simulink model "CS637Assignment1_1"  (R2022a)
settings: Solver=VariableStepAuto  StartTime=0.0  StopTime=10.0  RelTol=1e-3
settings Model: Creator=kaush  LastModifiedBy=kaush

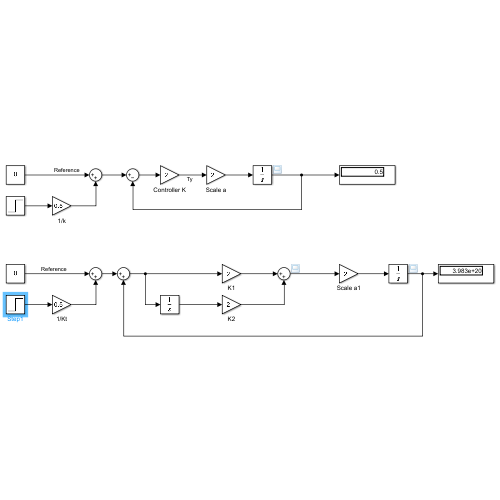
[thumbnail: Simulink's stored preview of the top-level diagram]
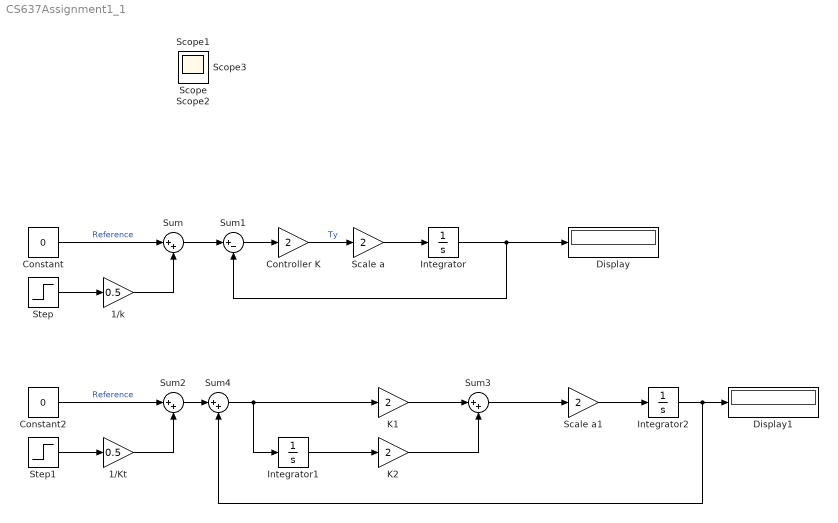
== system CS637Assignment1_1 ==
  1/Kt : Gain  Gain=0.5
  1/k : Gain  Gain=0.5
  Constant : Constant  Value=0
  Constant2 : Constant  Value=0
  Controller K : Gain  Gain=2
  Display : Display
  Display1 : Display
  Integrator : Integrator
  Integrator1 : Integrator
  Integrator2 : Integrator
  K1 : Gain  Gain=2
  K2 : Gain  Gain=2
  Scale a : Gain  Gain=2
  Scale a1 : Gain  Gain=2
  Step : Step  Time=0  SampleTime=0
  Step1 : Step  Time=0  SampleTime=0
  Sum{,2..4} (4 alike) : Sum  Inputs=|++
  Sum1 : Sum  Inputs=|+-
  Scope{,1..3} (4 alike) : Scope
  wires:
  1/k/1 -> Sum/2
  Constant/1 -> Sum/1  "Reference"
  Sum/1 -> Sum1/1
  Sum1/1 -> Controller K/1
  Controller K/1 -> Scale a/1  "Ty"
  Scale a/1 -> Integrator/1
  Integrator/1 -> Display/1, Sum1/2
  Step/1 -> 1/k/1
  Step1/1 -> 1/Kt/1
  Constant2/1 -> Sum2/1  "Reference"
  1/Kt/1 -> Sum2/2
  Integrator1/1 -> K2/1
  K2/1 -> Sum3/2
  K1/1 -> Sum3/1
  Sum3/1 -> Scale a1/1
  Scale a1/1 -> Integrator2/1
  Sum2/1 -> Sum4/1
  Sum4/1 -> K1/1, Integrator1/1
  Integrator2/1 -> Display1/1, Sum4/2
